simulink model "PID_controller"  (R2015b)
settings: Solver=VariableStepAuto  StartTime=0.0  StopTime=10.0  RelTol=1e-3
values from neighbouring files (symbols this model uses):
  c = 0    [NonLinearAnalysis.m]    (also in Run_Delta_R_Sim.m; analyse_lin_dynamics.m; analyse_steadystate.m; analyse_ulin_dynamics kopi.m)
  Kd_r = 0    [headingController.m]
  Ki_r = 0    [headingController.m]
  Kp_r = 1    [headingController.m]
  N = 0.1    [headingController.m]
  psi0 = 0    [NonLinearAnalysis.m]    (also in Run_Delta_R_Sim.m; analyse_lin_dynamics.m; analyse_steadystate.m; analyse_ulin_dynamics kopi.m)
  r0 = 0    [NonLinearAnalysis.m]    (also in Run_Delta_R_Sim.m; analyse_lin_dynamics.m; analyse_steadystate.m; analyse_ulin_dynamics kopi.m)
  tsamp = 10    [NonLinearAnalysis.m]    (also in analyse_lin_dynamics.m; analyse_steadystate.m; analyse_ulin_dynamics kopi.m; analyse_ulin_dynamics.m)
  v0 = [6.63 0]'    [NonLinearAnalysis.m]    (also in Run_Delta_R_Sim.m; analyse_lin_dynamics.m; analyse_steadystate.m; analyse_ulin_dynamics kopi.m)
undefined symbols (not defined in the file or in its folder): msfartoystyring
undefined symbols (not defined in the file): p0
settings Model: Creator=ShivJeet  LastModifiedBy=ShivJeet

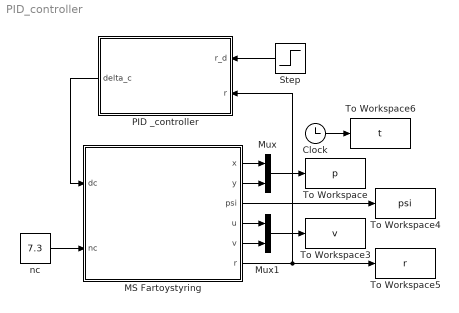
== system PID_controller ==
  Clock : Clock
  MS Fartoystyring : Subsystem  mask(MS Fartoystyring for Assignment 3 G&C){x0=p0(1), y0=p0(2), u0=v0(1), v0=v0(2), psi0=psi0, r0=r0, c=c}
      mask prompts: x0 "x(t0) (m)"; y0 "y(t0) (m)"; u0 "u(t0) (m/s)"; v0 "v(t0) (m/s)"; psi0 "psi(t0) (rad)"; r0 "r(t0) (rad/s)"; c "current (0 or 1)"
      mask help:
      | Block corresponding to Figure 1 in the assignment text. Gives the response of the ship.
      |
      | The design speed of MS Fartoystyring is u=8.23 m/s.
      |
      | Input:
      | dc: commanded rudder (rad), dmax=25*pi/180
      | nc: commanded shaft speed (rad/s), nmax=85*2*pi/60
      |
      | Output:
      | x: north pos (m)
      | y: east pos (m)
      | u: surge (m/s)
      | v: sway (m/s)
      | psi: heading (rad)
      | r: yaw (rad/s)
      mask Help: Comments, bugs and help requests can be directed to the TA. Email on course website.
  Mux : Mux  Inputs=2
  Mux1 : Mux  Inputs=2
  PID _controller : Subsystem
  Step : Step  SampleTime=0
  To Workspace : ToWorkspace  VariableName=p  SampleTime=tsamp
  To Workspace3 : ToWorkspace  VariableName=v  SampleTime=tsamp
  To Workspace4 : ToWorkspace  VariableName=psi  SampleTime=tsamp
  To Workspace5 : ToWorkspace  VariableName=r  SampleTime=tsamp
  To Workspace6 : ToWorkspace  VariableName=t  SampleTime=tsamp
  nc : Constant  Value=7.3
  wires:
  Clock/1 -> To Workspace6/1
  MS Fartoystyring/1(x) -> Mux/1
  MS Fartoystyring/2(y) -> Mux/2
  MS Fartoystyring/4(u) -> Mux1/1
  MS Fartoystyring/5(v) -> Mux1/2
  Mux/1 -> To Workspace/1
  Mux1/1 -> To Workspace3/1
  MS Fartoystyring/3(psi) -> To Workspace4/1
  MS Fartoystyring/6(r) -> PID _controller/2(r), To Workspace5/1
  nc/1 -> MS Fartoystyring/2(nc)
  PID _controller/1(delta_c) -> MS Fartoystyring/1(dc)
  Step/1 -> PID _controller/1(r_d)

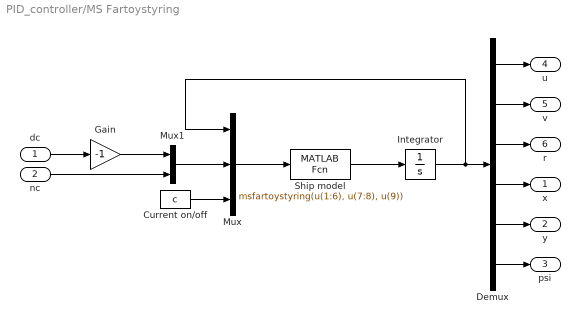
== system PID_controller/MS Fartoystyring ==
  dc : Inport
  nc : Inport  Port=2
  Current on/off : Constant  Value=c
  Demux : Demux  Outputs=6
  Gain : Gain  Gain=-1
  Integrator : Integrator  InitialCondition=[u0 v0 r0 x0 y0 psi0]'
  Mux : Mux  Inputs=3
  Mux1 : Mux  Inputs=2
  Ship model : MATLABFcn  MATLABFcn=msfartoystyring(u(1:6), u(7:8), u(9))  OutputDimensions=6
  x : Outport
  y : Outport  Port=2
  psi : Outport  Port=3
  u : Outport  Port=4
  v : Outport  Port=5
  r : Outport  Port=6
  wires:
  Integrator/1 -> Mux/1, Demux/1
  Mux1/1 -> Mux/2
  dc/1 -> Gain/1
  nc/1 -> Mux1/2
  Demux/1 -> u/1
  Demux/2 -> v/1
  Demux/3 -> r/1
  Demux/4 -> x/1
  Demux/5 -> y/1
  Demux/6 -> psi/1
  Current on/off/1 -> Mux/3
  Ship model/1 -> Integrator/1
  Mux/1 -> Ship model/1
  Gain/1 -> Mux1/1

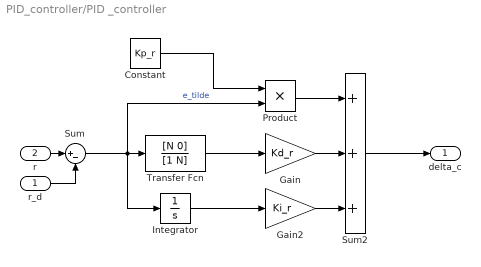
== system PID_controller/PID _controller ==
  r_d : Inport
  r : Inport  Port=2
  Constant : Constant  Value=Kp_r
  Gain : Gain  Gain=Kd_r
  Gain2 : Gain  Gain=Ki_r
  Integrator : Integrator
  Product : Product
  Sum : Sum  Inputs=|+-
  Sum2 : Sum  Inputs=+++
  Transfer Fcn : TransferFcn  Numerator=[N 0]  Denominator=[1 N]
  delta_c : Outport
  wires:
  r/1 -> Sum/1
  r_d/1 -> Sum/2
  Sum/1 -> Integrator/1, Product/2, Transfer Fcn/1  "e_tilde"
  Gain/1 -> Sum2/2
  Transfer Fcn/1 -> Gain/1
  Product/1 -> Sum2/1
  Integrator/1 -> Gain2/1
  Gain2/1 -> Sum2/3
  Sum2/1 -> delta_c/1
  Constant/1 -> Product/1
